simulink model "Solar_za_naponski"  (R2023b)
settings: Solver=FixedStepAuto  StartTime=0.0  StopTime=7.1  FixedStep=1e-4  RelTol=1e-3
undefined symbols (not defined in the file): pv_data, pv_eq, pv_in
libraries: simulink x1
settings Model: Creator=teo  LastModifiedBy=teo

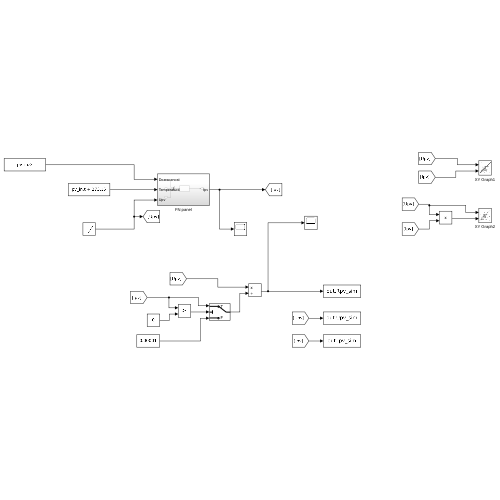
[thumbnail: Simulink's stored preview of the top-level diagram]
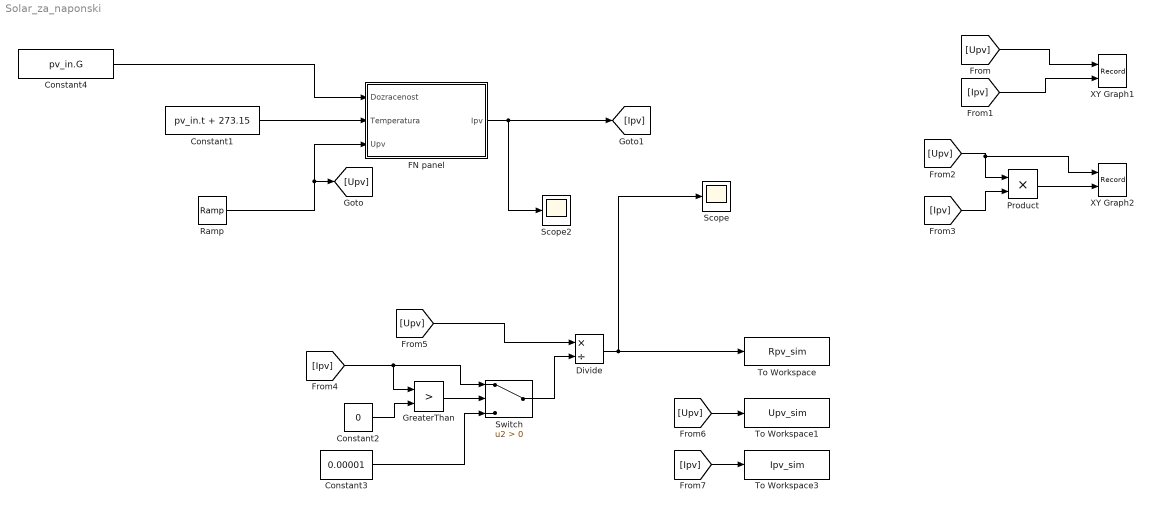
== system Solar_za_naponski ==
  Constant1 : Constant  Value=pv_in.t + 273.15
  Constant2 : Constant  Value=0
  Constant3 : Constant  Value=0.00001
  Constant4 : Constant  Value=pv_in.G
  Divide : Product  Inputs=*/
  FN panel : Subsystem
  GreaterThan : RelationalOperator  Operator=>  OutDataTypeStr=boolean  RndMeth=Simplest  InputSameDT=off
  Product : Product
  Ramp : simulink/Sources/Ramp  slope=1  start=0  InitialOutput=0
  Scope : Scope
  Scope2 : Scope
  Switch : Switch  Criteria=u2 > Threshold  SaturateOnIntegerOverflow=off  InputSameDT=off
  To Workspace : ToWorkspace  VariableName=Rpv_sim  SaveFormat=Timeseries  SampleTime=-1
  To Workspace1 : ToWorkspace  VariableName=Upv_sim  SaveFormat=Timeseries  SampleTime=-1
  To Workspace3 : ToWorkspace  VariableName=Ipv_sim  SaveFormat=Timeseries  SampleTime=-1
  XY Graph1 : Record  FileSettingsInternal="{\"entries\":[{\"content\":{\"excelSettings\":{\"content\":{},\"type\":\"Streamout.ExcelSettings\"}},\"type\":\"Streamout.FileSettingStorage\",\"uuid\":\"\"}],\"packageUris\":[\"http:\\/\\/schema.mathworks.com\\/mf0\\/streamout_blocks\\/R2020a\"],\"version\":\"1.0\"}"  Layout=[1 1]  SignalsInternal="{\"entries\":[{\"content\":{\"signals\":[{\"content\":{\"blockPath\":[],\"dimensions\":[1],\"domain\":\"\",\"lineColor\":\"#edb120\",\"plots\":[1],\"port\":1,\"sid\":[\"\"],\"signalID\":10577,\"signalName\":\"From\"},\"type\":\"RecordBlkView.Signal\",\"uuid\":\"\"},{\"content\":{\"blockPath\":[],\"dimensions\":[1],\"domain\":\"\",\"lineColor\":\"#7e2f8e\",\"plots\":[1],\"port\":2,\"sid\":[\"\"],\"signalID\":10581,\"signalName\":\"From1\"},\"type\":\"RecordBlkView.Signal\",\"uuid\":\"\"}]},\"type\":\"RecordBlkView.InputSignals\",\"uuid\":\"\"}],\"packageUris\":[\"http:\\/\\/schema.mathworks.com\\/mf0\\/streamout_blocks\\/R2020a\"],\"version\":\"1.0\"}"  VisualizationBindings="{\"xyplotplugin\":{\"info\":[{\"series\":[{\"bindingParametersList\":[{\"parameter\":\"X-Axis\",\"signalID\":10577,\"signalName\":\"From\"},{\"parameter\":\"Y-Axis\",\"signalID\":10581,\"signalName\":\"From1\"}],\"seriesID\":9702},{\"bindingParametersList\":[{\"parameter\":\"X-Axis\",\"signalID\":10577,\"signalName\":\"From\"},{\"parameter\":\"Y-Axis\",\"signalID\":10581,\"signalName\":\"From1\"}],\"seriesID\":41395}],\"subplotID\":1}]}}"  CompatibilityTag=XY  st=-1
  XY Graph2 : Record  VariableName=PV_record  Filename=Solar_800W.mldatx  FileSettingsInternal="{\"entries\":[{\"content\":{\"excelSettings\":{\"content\":{},\"type\":\"Streamout.ExcelSettings\"}},\"type\":\"Streamout.FileSettingStorage\",\"uuid\":\"\"}],\"packageUris\":[\"http:\\/\\/schema.mathworks.com\\/mf0\\/streamout_blocks\\/R2020a\"],\"version\":\"1.0\"}"  Layout=[1 1]  SignalsInternal="{\"entries\":[{\"content\":{\"signals\":[{\"content\":{\"blockPath\":[],\"dimensions\":[1],\"domain\":\"\",\"lineColor\":\"#77ac30\",\"plots\":[1],\"port\":1,\"sid\":[\"\"],\"signalID\":10585,\"signalName\":\"From2\"},\"type\":\"RecordBlkView.Signal\",\"uuid\":\"\"},{\"content\":{\"blockPath\":[],\"dimensions\":[1],\"domain\":\"\",\"lineColor\":\"#4dbeee\",\"plots\":[1],\"port\":2,\"sid\":[\"\"],\"signalID\":10589,\"signalName\":\"Product\"},\"type\":\"RecordBlkView.Signal\",\"uuid\":\"\"}]},\"type\":\"RecordBlkView.InputSignals\",\"uuid\":\"\"}],\"packageUris\":[\"http:\\/\\/schema.mathworks.com\\/mf0\\/streamout_blocks\\/R2020a\"],\"version\":\"1.0\"}"  VisualizationBindings="{\"xyplotplugin\":{\"info\":[{\"series\":[{\"bindingParametersList\":[{\"parameter\":\"X-Axis\",\"signalID\":10585,\"signalName\":\"From2\"},{\"parameter\":\"Y-Axis\",\"signalID\":10589,\"signalName\":\"Product\"}],\"seriesID\":28985}],\"subplotID\":1}]}}"  CompatibilityTag=XY  st=-1
  wires:
  [Upv] -> XY Graph1/1
  [Ipv] -> XY Graph1/2
  [Ipv] -> Product/2
  FN panel/1(Ipv) -> [Ipv], Scope2/1
  Ramp/1 -> [Upv], FN panel/3(Upv)
  Product/1 -> XY Graph2/2
  [Upv] -> XY Graph2/1, Product/1
  Divide/1 -> Scope/1, To Workspace/1
  [Ipv] -> GreaterThan/1, Switch/1
  Switch/1 -> Divide/2
  [Upv] -> Divide/1
  GreaterThan/1 -> Switch/2
  Constant2/1 -> GreaterThan/2
  Constant3/1 -> Switch/3
  [Upv] -> To Workspace1/1
  [Ipv] -> To Workspace3/1
  Constant4/1 -> FN panel/1(Dozracenost)
  Constant1/1 -> FN panel/2(Temperatura)

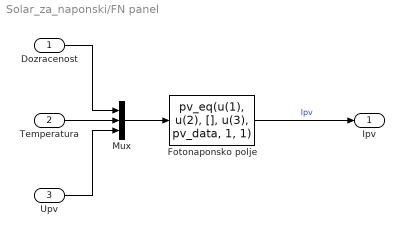
== system Solar_za_naponski/FN panel ==
  Dozracenost : Inport
  Temperatura : Inport  Port=2
  Upv : Inport  Port=3
  Fotonaponsko polje : MATLABFcn  MATLABFcn=pv_eq(u(1), u(2), [], u(3), pv_data, 1, 1)  OutputDimensions=1
  Mux : Mux  Inputs=3
  Ipv : Outport
  wires:
  Fotonaponsko polje/1 -> Ipv/1  "Ipv"
  Mux/1 -> Fotonaponsko polje/1
  Dozracenost/1 -> Mux/1
  Temperatura/1 -> Mux/2
  Upv/1 -> Mux/3
